simulink model "ADC_reader_simulink"  (R2025a)
settings: Solver=FixedStepAuto  StartTime=0.0  StopTime=inf  FixedStep=0.01  RelTol=1e-3  EnableMultiTasking=on
libraries: stm32f4xxblockslib x8
settings Model: STM32="{\"AnalogInput\":[{\"ID\":\"test_poten:20\"},{\"ID\":\"test_poten:28\"},{\"ID\":\"ADC_reader:28\"},{\"ID\":\"ADC_reader:20\"},{\"ID\":\"ADC_reader:14\"},{\"ID\":\"ADC_reader:11\"},{\"ID\":\"ADC_reader:8\"},{\"ID\":\"ADC_reader:5\"},{\"ID\":\"ADC_reader:1\"},{\"ID\":\"ADC_reader_simulink:14\"},{\"ID\":\"ADC_reader_simulink:11\"},{\"ID\":\"ADC_reader_simulink:8\"},{\"ID\":\"ADC_reader_simulink:5\"},{\"ID\":\"ADC_reader_simulink:1\"},{\"ID\":\"ADC_reader_simulink:20\"}]}"  Creator=ioonz  LastModifiedBy=Acer
settings OptimizationCC: DefaultParameterBehavior=Inlined  EnhancedBackFolding=on  PassReuseOutputArgsAs=Individual arguments  ZeroExternalMemoryAtStartup=off  ZeroInternalMemoryAtStartup=off  MaxStackSize=512  OptimizeBlockOrder=speed  DifferentSizesBufferReuse=on  OptimizationCustomize=off  EfficientTunableParamExpr=on
settings DebuggingCC: ParameterTunabilityLossMsg=error
settings HardwareCC: ProdBitPerPointer=32.0  ProdBitPerSizeT=32.0  ProdBitPerPtrDiffT=32.0  ProdLargestAtomicInteger=Long  ProdLargestAtomicFloat=Double  ProdWordSize=32.0  ProdLongLongMode=on  ProdHWDeviceType=ARM Compatible->ARM Cortex-M
settings SFSimCC: MATLABDynamicMemAlloc=off
settings RTWCC: SystemTargetFile=ert.tlc  HardwareBoard=STM32G4xx Based  TemplateMakefile=ert_default_tmf  Toolchain=GNU Tools for ARM Embedded Processors  Description=Embedded Coder
settings CodeAppCC: ForceParamTrailComments=on  IgnoreCustomStorageClasses=off  OperatorAnnotations=on  SimulinkDataObjDesc=on  SFDataObjDesc=on  InsertBlockDesc=on
settings ERTTargetCC: ExtModeTransport=3.0  ExtModeStaticAllocSize=2048.0  TargetLangStandard=C99 (ISO)  CodeReplacementLibrary=ARM Cortex-M

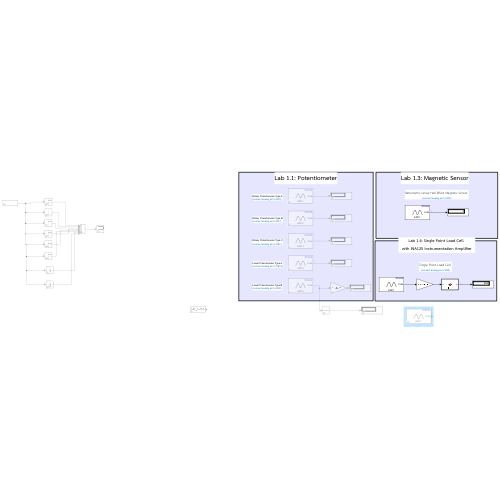
[thumbnail: Simulink's stored preview of the top-level diagram]
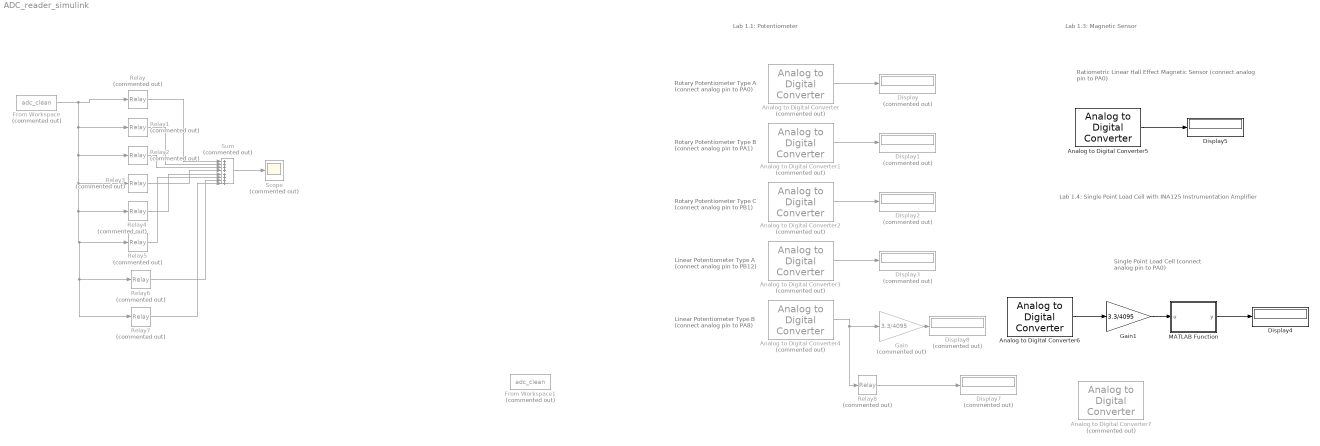
== system ADC_reader_simulink ==
  note: Lab 1.1: Potentiometer
  note: Rotary Potentiometer Type A
      | (connect analog pin to PA0)
  note: Rotary Potentiometer Type B
      | (connect analog pin to PA1)
  note: Rotary Potentiometer Type C
      | (connect analog pin to PB1)
  note: Linear Potentiometer Type A
      | (connect analog pin to PB12)
  note: Linear Potentiometer Type B
      | (connect analog pin to PA8)
  note: Ratiometric Linear Hall Effect Magnetic Sensor
      | (connect analog pin to PA0)
  note: Single Point Load Cell
      | (connect analog pin to PA0)
  note: Lab 1.3: Magnetic Sensor
  note: Lab 1.4: Single Point Load Cell
      | with INA125 Instrumentation Amplifier
  Analog to Digital Converter : stm32f4xxblockslib/Analog to Digital Converter  Commented=on  ADCModule=ADC1  ConversionGroup=Regular  TriggerMode=Trigger and read  NumberOfConversions=1  EnableBufferConv=off  BufferLength=1  OutputStatus=off  SampleTime=-1  EnableSimPort=off  hoistedMaskSrc=ECSoC/ECSimCodegen/Analog to Digital Converter
  Analog to Digital Converter1 : stm32f4xxblockslib/Analog to Digital Converter  Commented=on  ADCModule=ADC2  ConversionGroup=Regular  TriggerMode=Trigger and read  NumberOfConversions=1  EnableBufferConv=off  BufferLength=1  OutputStatus=off  SampleTime=-1  EnableSimPort=off  hoistedMaskSrc=ECSoC/ECSimCodegen/Analog to Digital Converter
  Analog to Digital Converter2 : stm32f4xxblockslib/Analog to Digital Converter  Commented=on  ADCModule=ADC3  ConversionGroup=Regular  TriggerMode=Trigger and read  NumberOfConversions=1  EnableBufferConv=off  BufferLength=1  OutputStatus=off  SampleTime=-1  EnableSimPort=off  hoistedMaskSrc=ECSoC/ECSimCodegen/Analog to Digital Converter
  Analog to Digital Converter3 : stm32f4xxblockslib/Analog to Digital Converter  Commented=on  ADCModule=ADC4  ConversionGroup=Regular  TriggerMode=Trigger and read  NumberOfConversions=1  EnableBufferConv=off  BufferLength=1  OutputStatus=off  SampleTime=-1  EnableSimPort=off  hoistedMaskSrc=ECSoC/ECSimCodegen/Analog to Digital Converter
  Analog to Digital Converter4 : stm32f4xxblockslib/Analog to Digital Converter  Commented=on  ADCModule=ADC5  ConversionGroup=Regular  TriggerMode=Trigger and read  NumberOfConversions=1  EnableBufferConv=off  BufferLength=1  OutputStatus=off  SampleTime=-1  EnableSimPort=off  hoistedMaskSrc=ECSoC/ECSimCodegen/Analog to Digital Converter
  Analog to Digital Converter5 : stm32f4xxblockslib/Analog to Digital Converter  ADCModule=ADC1  ConversionGroup=Regular  TriggerMode=Trigger and read  NumberOfConversions=1  EnableBufferConv=off  BufferLength=1  OutputStatus=off  SampleTime=-1  EnableSimPort=off  hoistedMaskSrc=ECSoC/ECSimCodegen/Analog to Digital Converter
  Analog to Digital Converter6 : stm32f4xxblockslib/Analog to Digital Converter  ADCModule=ADC1  ConversionGroup=Regular  TriggerMode=Trigger and read  NumberOfConversions=1  EnableBufferConv=off  BufferLength=1  OutputStatus=off  SampleTime=-1  EnableSimPort=off  hoistedMaskSrc=ECSoC/ECSimCodegen/Analog to Digital Converter
  Analog to Digital Converter7 : stm32f4xxblockslib/Analog to Digital Converter  Commented=on  ADCModule=ADC1  ConversionGroup=Regular  TriggerMode=Trigger and read  NumberOfConversions=1  EnableBufferConv=off  BufferLength=1  OutputStatus=off  SampleTime=-1  EnableSimPort=off  hoistedMaskSrc=ECSoC/ECSimCodegen/Analog to Digital Converter
  Display{,1..3,7..8} (6 alike) : Display  Commented=on
  Display4 : Display
  Display5 : Display
  From Workspace : FromWorkspace  Commented=on  VariableName=adc_clean
  From Workspace1 : FromWorkspace  Commented=on  VariableName=adc_clean
  Gain : Gain  Commented=on  Gain=3.3/4095
  Gain1 : Gain  Gain=3.3/4095
  MATLAB Function : MATLAB Function  TreatAsAtomicUnit=on
  Relay : Relay  Commented=on  OnSwitchValue=44  OffSwitchValue=0
  Relay1 : Relay  Commented=on  OnSwitchValue=117  OffSwitchValue=44
  Relay2 : Relay  Commented=on  OnSwitchValue=236  OffSwitchValue=117
  Relay3 : Relay  Commented=on  OnSwitchValue=1114  OffSwitchValue=236
  Relay4 : Relay  Commented=on  OnSwitchValue=1868  OffSwitchValue=1114
  Relay5 : Relay  Commented=on  OnSwitchValue=2650  OffSwitchValue=1868
  Relay6 : Relay  Commented=on  OnSwitchValue=3528  OffSwitchValue=2650
  Relay7 : Relay  Commented=on  OnSwitchValue=4045  OffSwitchValue=3528
  Relay8 : Relay  Commented=on  OnSwitchValue=2866.5  OffSwitchValue=1023.75
  Scope : Scope  Commented=on
      settings: ActiveDisplayYMinimum=-9.9498138518834143  ActiveDisplayYMaximum=23.913735557110503
  Sum : Sum  Commented=on  Inputs=|++++++++
  wires:
  Analog to Digital Converter/1 -> Display/1
  Analog to Digital Converter1/1 -> Display1/1
  Analog to Digital Converter2/1 -> Display2/1
  Analog to Digital Converter3/1 -> Display3/1
  Analog to Digital Converter4/1 -> Gain/1, Relay8/1
  Analog to Digital Converter5/1 -> Display5/1
  From Workspace/1 -> Relay7/1, Relay6/1, Relay5/1, Relay4/1, Relay3/1, Relay2/1, Relay1/1, Relay/1
  Relay/1 -> Sum/1
  Relay1/1 -> Sum/2
  Relay2/1 -> Sum/3
  Relay3/1 -> Sum/4
  Relay4/1 -> Sum/5
  Relay5/1 -> Sum/6
  Relay6/1 -> Sum/7
  Relay7/1 -> Sum/8
  Sum/1 -> Scope/1
  Relay8/1 -> Display7/1
  Gain/1 -> Display8/1
  Analog to Digital Converter6/1 -> Gain1/1
  Gain1/1 -> MATLAB Function/1(u)
  MATLAB Function/1(y) -> Display4/1

== matlab function ADC_reader_simulink/MATLAB Function ==
  data: u input; y output
function y = fcn(u)

y =(-196.34*(u^6)) + 1638.6*(u^5) - 5279.2*(u^4) + 8270.1*(u^3) - 6493.7*(u^2) + 6201.3*u + 67.315;
